simulink model "Simulation"  (R2024a)
settings: Solver=VariableStepAuto  StartTime=0.0  StopTime=10.0  RelTol=1e-3
settings Model: Creator=daced  LastModifiedBy=daced

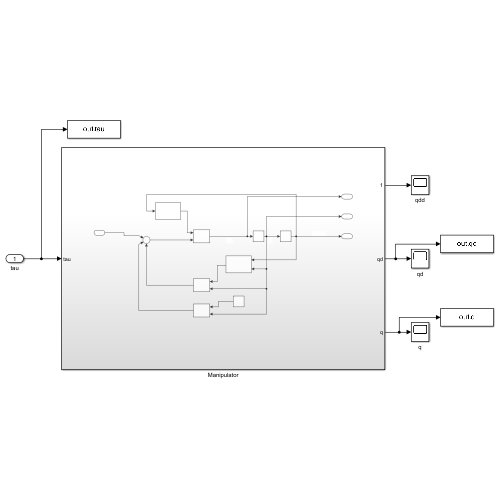
[thumbnail: Simulink's stored preview of the top-level diagram]
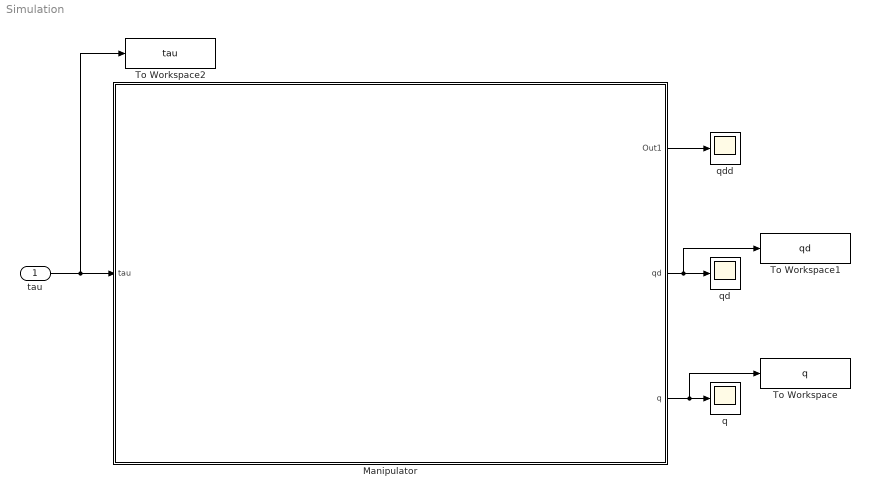
== system Simulation ==
  tau : Inport
  Manipulator : Subsystem
  To Workspace : ToWorkspace  VariableName=q  SaveFormat=Timeseries  SampleTime=-1
  To Workspace1 : ToWorkspace  VariableName=qd  SaveFormat=Timeseries  SampleTime=-1
  To Workspace2 : ToWorkspace  VariableName=tau  SaveFormat=Timeseries  SampleTime=-1
  q : Scope
  qd : Scope
  qdd : Scope
  wires:
  tau/1 -> To Workspace2/1, Manipulator/1(tau)
  Manipulator/1(Out1) -> qdd/1
  Manipulator/2(qd) -> To Workspace1/1, qd/1
  Manipulator/3(q) -> To Workspace/1, q/1

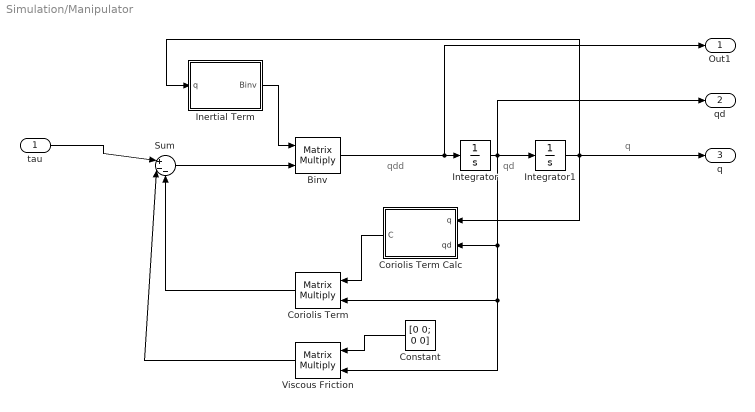
== system Simulation/Manipulator ==
  note: q
  note: qd
  note: qdd
  tau : Inport
  Binv : Product  Multiplication=Matrix(*)
  Constant : Constant  Value=[0 0; 0 0]
  Coriolis Term : Product  Multiplication=Matrix(*)
  Coriolis Term Calc : MATLAB Function  TreatAsAtomicUnit=on
  Inertial Term : MATLAB Function  TreatAsAtomicUnit=on
  Integrator : Integrator  InitialCondition=[0;0]
  Integrator1 : Integrator  InitialCondition=[0;0]
  Sum : Sum  Inputs=|+--
  Viscous Friction : Product  Multiplication=Matrix(*)
  Out1 : Outport
  qd : Outport  Port=2
  q : Outport  Port=3
  wires:
  Coriolis Term Calc/1(C) -> Coriolis Term/1
  Coriolis Term/1 -> Sum/3
  Integrator/1 -> qd/1, Viscous Friction/2, Coriolis Term/2, Coriolis Term Calc/2(qd), Integrator1/1
  Binv/1 -> Out1/1, Integrator/1
  Integrator1/1 -> Coriolis Term Calc/1(q), q/1, Inertial Term/1(q)
  Sum/1 -> Binv/2
  Inertial Term/1(Binv) -> Binv/1
  Constant/1 -> Viscous Friction/1
  Viscous Friction/1 -> Sum/2
  tau/1 -> Sum/1

== matlab function Simulation/Manipulator/Inertial Term ==
  data: q input; Binv output
function Binv = Binv(q)
% calculate inertial term
% Bfcn should be preexistng function in directory
% q = [th1; th2]
B = Bfcn(q(1), q(2));
Binv = inv(B);

== matlab function Simulation/Manipulator/Coriolis Term Calc ==
  data: q input; C output; qd input
function C = C(q, qd)
% calculates Christoffel term
% Cfcnn from preexisting function in directory
% q = [th1 th2], qd = [th1d th2d]
C = Cfcn(q(1), q(2), qd(1), qd(2));
